simulink model "FMS"  (R2025a)
settings: Solver=VariableStepAuto  StartTime=0.0  StopTime=500  RelTol=1e-3
libraries: simulink x2
settings Model: Creator=ramch  LastModifiedBy=ramch

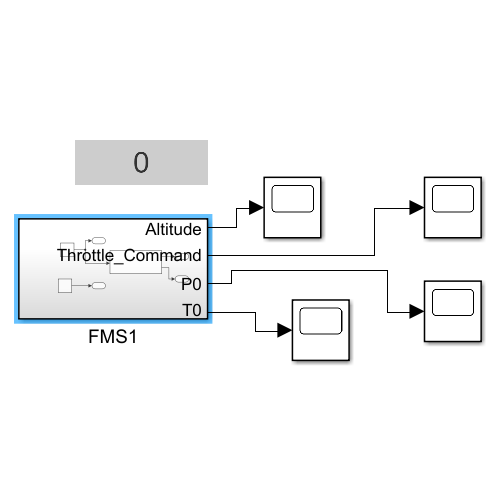
[thumbnail: Simulink's stored preview of the top-level diagram]
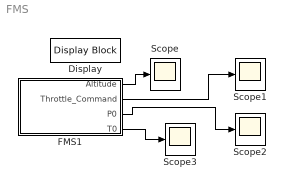
== system FMS ==
  Display : DisplayBlock  LabelPosition=Hide  Transparency=1  GridColor=[0.502, 0.502, 0.502]
  FMS1 : Subsystem
  Scope{,1..3} (4 alike) : Scope
      Scope settings: ActiveDisplayYMinimum=-1  ActiveDisplayYMaximum=1
      Scope1 settings: ActiveDisplayYMinimum=0.2125  ActiveDisplayYMaximum=1.0875
      Scope2 settings: ActiveDisplayYMinimum=94327.842367227786  ActiveDisplayYMaximum=103419.2768689892  DataLoggingVariableName=ScopeData2
      Scope3 settings: ActiveDisplayYMinimum=-1  ActiveDisplayYMaximum=1  DataLoggingVariableName=ScopeData3
  wires:
  FMS1/1(Altitude) -> Scope/1
  FMS1/4(T0) -> Scope3/1
  FMS1/2(Throttle_Command) -> Scope1/1
  FMS1/3(P0) -> Scope2/1

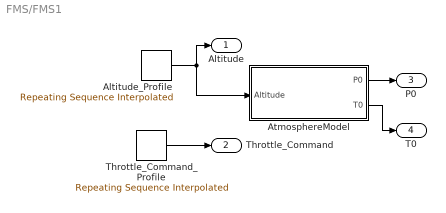
== system FMS/FMS1 ==
  Altitude_Profile : simulink/Sources/Repeating Sequence Interpolated  OutValues=[0 1500 6000 10000 10000 5000 0]  TimeValues=[0 50 100 200 300 400 500]  LookUpMeth=Interpolation-Use End Values  tsamp=0.1  OutMin=[]  OutMax=[]  OutDataTypeStr=double  OutputDataTypeScalingMode=double  OutDataType=fixdt(0,8)  OutScaling=2^-10
  AtmosphereModel : MATLAB Function  TreatAsAtomicUnit=on
  Throttle_Command_Profile : simulink/Sources/Repeating Sequence Interpolated  OutValues=[1.0 0.9 0.7 0.5 0.5 0.6 0.3]  TimeValues=[0 50 100 200 300 400 500]  LookUpMeth=Use Input Below  tsamp=0.1  OutMin=[]  OutMax=[]  OutDataTypeStr=double  OutputDataTypeScalingMode=double  OutDataType=fixdt(0,8)  OutScaling=2^-10
  Altitude : Outport
  Throttle_Command : Outport  Port=2
  P0 : Outport  Port=3
  T0 : Outport  Port=4
  wires:
  AtmosphereModel/1(P0) -> P0/1
  AtmosphereModel/2(T0) -> T0/1
  Altitude_Profile/1 -> AtmosphereModel/1(Altitude), Altitude/1
  Throttle_Command_Profile/1 -> Throttle_Command/1

== matlab function FMS/FMS1/AtmosphereModel ==
  data: Altitude input; P0 output; T0 output
function [P0, T0] = AtmosphereModel(Altitude)
% Calculates ambient pressure (P0) and temperature (T0) using ISA model

    T0_sea = 288.15;   % Sea level temperature (K)
    P0_sea = 101325;   % Sea level pressure (Pa)
    L = 0.0065;        % Lapse rate (K/m)
    R = 287.05;        % Gas constant (J/kg·K)
    g = 9.80665;       % Gravity (m/s²)

    if Altitude < 11000
        T0 = T0_sea - L * Altitude;
        P0 = P0_sea * (1 - (L * Altitude) / T0_sea)^(g / (R * L));
    else
        T0 = 216.65;
        P11 = P0_sea * (1 - (L * 11000) / T0_sea)^(g / (R * L));
        P0 = P11 * exp(-g * (Altitude - 11000) / (R * T0));
    end
end
